simulink model "crc_8_optimized"  (R2021b)
settings: Solver=FixedStepDiscrete  StartTime=0.0  StopTime=inf  FixedStep=0.01  RelTol=1e-3
libraries: commcrc2 x1
settings Model: Creator=jekyll  LastModifiedBy=jekyll
settings OptimizationCC: DefaultParameterBehavior=Inlined  EnhancedBackFolding=on  PassReuseOutputArgsAs=Individual arguments  OptimizeBlockOrder=speed  DifferentSizesBufferReuse=on  OptimizationCustomize=off  EfficientTunableParamExpr=on
settings DebuggingCC: ParameterTunabilityLossMsg=error
settings SFSimCC: MATLABDynamicMemAlloc=off
settings RTWCC: Description=Embedded Coder  SystemTargetFile=ert.tlc  GenCodeOnly=on  TemplateMakefile=ert_default_tmf
settings CodeAppCC: ForceParamTrailComments=on  IgnoreCustomStorageClasses=off  OperatorAnnotations=on  SimulinkDataObjDesc=on  SFDataObjDesc=on  InsertBlockDesc=on
settings ERTTargetCC: TargetLangStandard=C99 (ISO)  GenerateSampleERTMain=on  SupportAbsoluteTime=off  CodeInterfacePackaging=Reusable function  SupportNonFinite=off  SupportComplex=off  InlinedParameterPlacement=NonHierarchical  ERTCustomFileTemplate=example_file_process.tlc

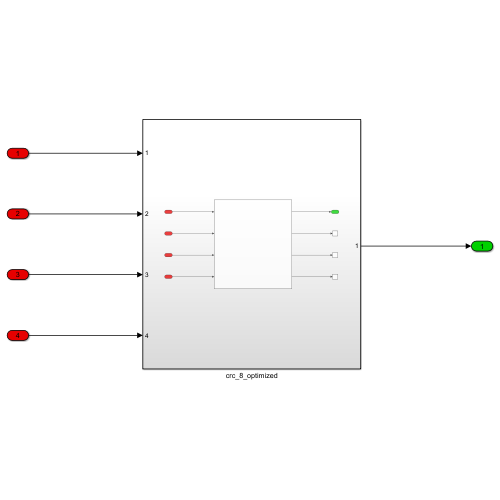
[thumbnail: Simulink's stored preview of the top-level diagram]
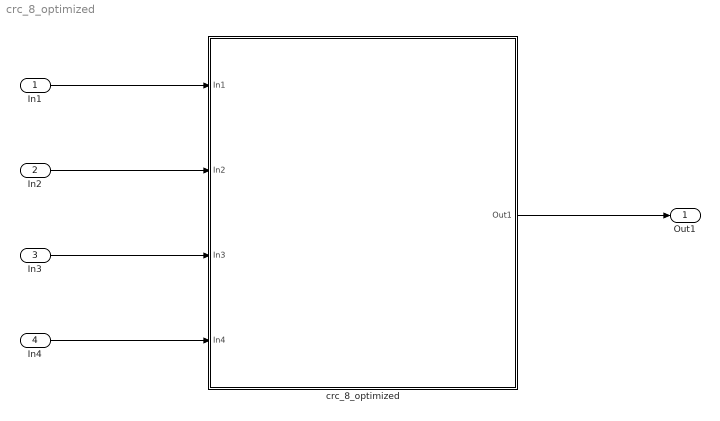
== system crc_8_optimized ==
  In1 : Inport  OutDataTypeStr=uint8
  In2 : Inport  Port=2  OutDataTypeStr=boolean
  In3 : Inport  Port=3  OutDataTypeStr=boolean
  In4 : Inport  Port=4  OutDataTypeStr=boolean
  crc_8_optimized : Subsystem
  Out1 : Outport  OutDataTypeStr=uint8
  wires:
  In1/1 -> crc_8_optimized/1(In1)
  In2/1 -> crc_8_optimized/2(In2)
  In3/1 -> crc_8_optimized/3(In3)
  In4/1 -> crc_8_optimized/4(In4)
  crc_8_optimized/1(Out1) -> Out1/1

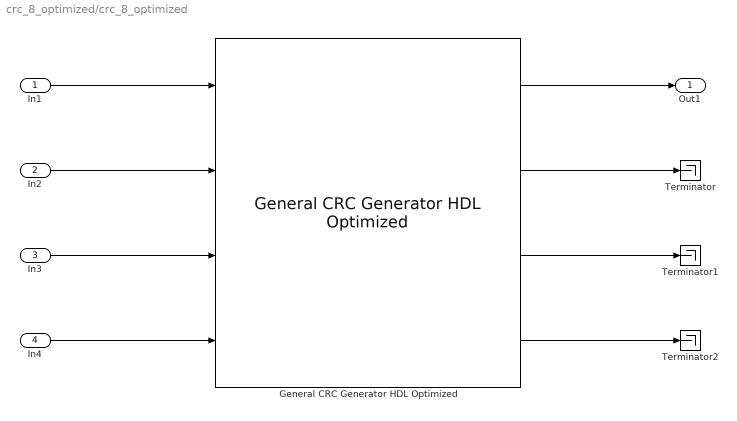
== system crc_8_optimized/crc_8_optimized ==
  In1 : Inport
  In2 : Inport  Port=2
  In3 : Inport  Port=3
  In4 : Inport  Port=4
  General CRC Generator HDL Optimized : commcrc2/General CRC Generator HDL Optimized  Polynomial=[1, 0, 0, 0, 1, 1, 1 , 0, 1]  InitialState=1  DirectMethod=on  ReflectInput=off  ReflectCRCChecksum=off  FinalXORValue=1  SimulateUsing=Code generation
      settings: SourceProductBaseCode=CM
  Terminator : Terminator
  Terminator1 : Terminator
  Terminator2 : Terminator
  Out1 : Outport
  wires:
  In4/1 -> General CRC Generator HDL Optimized/4
  In3/1 -> General CRC Generator HDL Optimized/3
  In1/1 -> General CRC Generator HDL Optimized/1
  In2/1 -> General CRC Generator HDL Optimized/2
  General CRC Generator HDL Optimized/1 -> Out1/1
  General CRC Generator HDL Optimized/2 -> Terminator/1
  General CRC Generator HDL Optimized/3 -> Terminator1/1
  General CRC Generator HDL Optimized/4 -> Terminator2/1
